simulink model "XYSim"  (R2023b)
settings: Solver=VariableStepAuto  StartTime=0.0  StopTime=30  RelTol=1e-3
undefined symbols (not defined in the file): robot
libraries: simulink_extras x2, slpidlib x1, simulink x1
settings Model: Creator=leand  LastModifiedBy=leand

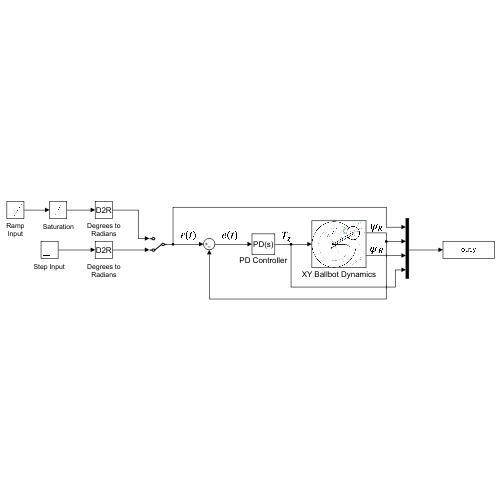
[thumbnail: Simulink's stored preview of the top-level diagram]
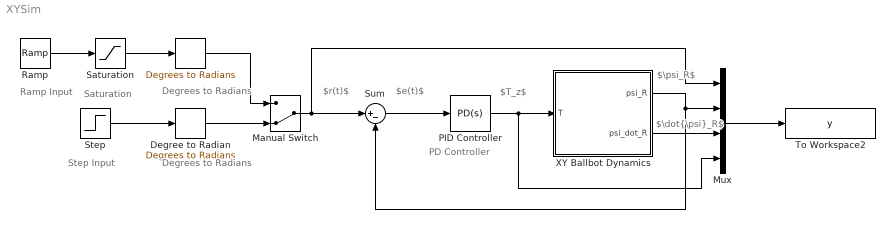
== system XYSim ==
  note: Step Input
  note: PD Controller
  note: Saturation
  note: Ramp
      | Input
  note: Degrees to
      | Radians
  note: $T_z$
  note: $r(t)$
  note: $e(t)$
  note: $\dot{\psi}_R$
  note: $\psi_R$
  note: Degrees to
      | Radians
  " " : simulink_extras/Transformations/Degrees to Radians
  Degree to Radian : simulink_extras/Transformations/Degrees to Radians
  Manual Switch : ManualSwitch  CurrentSetting=0
  Mux : Mux
  PID Controller : slpidlib/PID Controller  Controller=PD  Form=Parallel  TimeDomain=Continuous-time  UseExternalTs=off  SampleTime=-1  IntegratorMethod=Forward Euler  FilterMethod=Forward Euler  ControllerParametersSource=internal  P=-0.01  I=0  UseKiTs=off  D=-0.005  N=100  UseFilter=on  TunerSelectOption=Transfer Function Based (PID Tuner App)  InitialConditionSource=internal  InitialConditionForIntegrator=0  InitialConditionForFilter=0  DifferentiatorICPrevScaledInput=0  ExternalReset=none  TrackingMode=off  Kt=1  LimitOutput=off  SatLimitsSource=internal  UpperSaturationLimit=inf  LowerSaturationLimit=-inf  LinearizeAsGain=on  AntiWindupMode=none  Kb=1  LimitIntegrator=off  UpperIntegratorSaturationLimit=inf  LowerIntegratorSaturationLimit=-inf  POutMin=[]  POutMax=[]  IOutMin=[]  IOutMax=[]  DOutMin=[]  DOutMax=[]  NOutMin=[]  NOutMax=[]  SumOutMin=[]  SumOutMax=[]  SaturationOutMin=[]  SaturationOutMax=[]  PParamMin=[]  PParamMax=[]  IParamMin=[]  IParamMax=[]  DParamMin=[]  DParamMax=[]  NParamMin=[]  NParamMax=[]  KbParamMin=[]  KbParamMax=[]  KtParamMin=[]  KtParamMax=[]  KbOutMin=[]  KbOutMax=[]  KtOutMin=[]  KtOutMax=[]  IntegratorOutMin=[]  IntegratorOutMax=[]  FilterOutMin=[]  FilterOutMax=[]  SumI1OutMin=[]  SumI1OutMax=[]  SumI2OutMin=[]  SumI2OutMax=[]  SumI3OutMin=[]  SumI3OutMax=[]  SumI4OutMin=[]  SumI4OutMax=[]  SumDOutMin=[]  SumDOutMax=[]  DifferentiatorOutMin=[]  DifferentiatorOutMax=[]  FilterDiffOutCoefMin=[]  FilterDiffOutCoefMax=[]  ReciprocalOutMin=[]  ReciprocalOutMax=[]  SumDenOutMin=[]  SumDenOutMax=[]  SumNumOutMin=[]  SumNumOutMax=[]  DivideOutMin=[]  DivideOutMax=[]  UdiffTsProdOutMin=[]  UdiffTsProdOutMax=[]  NTsProdOutMin=[]  NTsProdOutMax=[]  UintegralTsProdOutMin=[]  UintegralTsProdOutMax=[]  UngainTsProdOutMin=[]  UngainTsProdOutMax=[]  ClampingZeroOutDataTypeStr=Inherit: Inherit via back propagation  ClampingZeroOutMin=[]  ClampingZeroOutMax=[]  FilterDenConstantOutDataTypeStr=Inherit: Inherit via back propagation  FilterDenConstantOutMin=[]  FilterDenConstantOutMax=[]  PCopyOutDataTypeStr=Inherit: Inherit via back propagation  PCopyOutMin=[]  PCopyOutMax=[]  NCopyOutDataTypeStr=Inherit: Inherit via back propagation  NCopyOutMin=[]  NCopyOutMax=[]  IntegratorContinuousStateAttributes=''  IntegratorStateMustResolveToSignalObject=off  IntegratorRTWStateStorageClass=Auto  FilterContinuousStateAttributes=''  FilterStateMustResolveToSignalObject=off  FilterRTWStateStorageClass=Auto  ParallelPVariant=InternalParameters  IdealPVariant=Disabled  IVariant=Disabled  DVariant=InternalParameters  IntegratorVariant=Disabled  SatVariant=Disabled  AWVariant=Disabled  PCopyVariant=Disabled  TRVariant=Disabled  FdbkBlocksVariant=Forward  IdealPFdbkVariant=Disabled  SatFdbkVariant=Disabled  DerivativeFilterVariant=ContFilter  NVariant=InternalParameters  NCopyVariant=Disabled  FilterICVariant=InternalICsFilter  IntegratorICVariant=Disabled  ExternalResetVariant=Disabled  TRSumVariant=Passthrough  SumFdbkVariant=Disabled  SumVariant=Sum_PD  TsampFilterVariant=InternalTs  TsampNgainVariant=Passthrough  TsampIntegralVariant=Disabled_SignalSpec  ExternalSaturationOutDataTypeStr=Inherit: Same as second input
  Ramp : simulink/Sources/Ramp  slope=15  start=0  InitialOutput=0
  Saturation : Saturate  UpperLimit=90  LowerLimit=0
  Step : Step  Time=0  After=15  SampleTime=0
  Sum : Sum  Inputs=|+-
  To Workspace2 : ToWorkspace  VariableName=y  SaveFormat=Timeseries  SampleTime=-1
  XY Ballbot Dynamics : Subsystem
      mask Display: image('XY.png');
  wires:
  XY Ballbot Dynamics/1(psi_R) -> Sum/2, Mux/2
  Sum/1 -> PID Controller/1
  PID Controller/1 -> Mux/4, XY Ballbot Dynamics/1(T)
  Ramp/1 -> Saturation/1
  Saturation/1 -> " "/1
  Manual Switch/1 -> Sum/1, Mux/1
  Step/1 -> Degree to Radian/1
  " "/1 -> Manual Switch/1
  Degree to Radian/1 -> Manual Switch/2
  Mux/1 -> To Workspace2/1
  XY Ballbot Dynamics/2(psi_dot_R) -> Mux/3

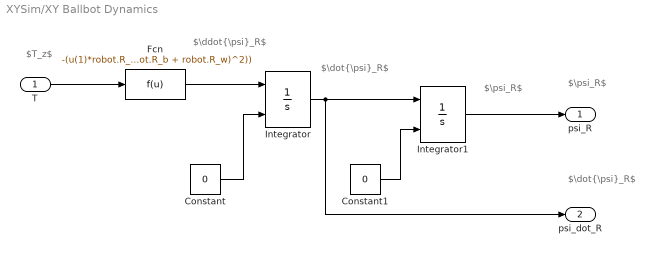
== system XYSim/XY Ballbot Dynamics ==
  note: $T_z$
  note: $\ddot{\psi}_R$
  note: $\dot{\psi}_R$
  note: $\psi_R$
  note: $\psi_R$
  note: $\dot{\psi}_R$
  T : Inport
  Constant : Constant  Value=0
  Constant1 : Constant  Value=0
  Fcn : Fcn  Expr=-(u(1)*robot.R_b)/(robot.R_w*(robot.I_r + robot.I_w + robot.m_w*(robot.R_b + robot.R_w)^2))
  Integrator : Integrator  InitialConditionSource=external
  Integrator1 : Integrator  InitialConditionSource=external
  psi_R : Outport
  psi_dot_R : Outport  Port=2
  wires:
  Constant/1 -> Integrator/2
  Integrator1/1 -> psi_R/1
  Integrator/1 -> Integrator1/1, psi_dot_R/1
  Constant1/1 -> Integrator1/2
  Fcn/1 -> Integrator/1
  T/1 -> Fcn/1
